simulink model "OrientationExample"  (R2024b)
settings: Solver=VariableStepAuto  StartTime=0.0  StopTime=inf  RelTol=1e-3
PostLoadFcn:
  | addpath(genpath(pwd))
settings Model: Creator=JesseJabezArendse  LastModifiedBy=JesseJabezArendse

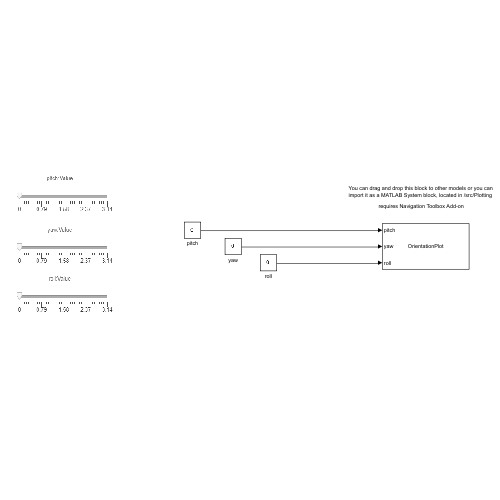
[thumbnail: Simulink's stored preview of the top-level diagram]
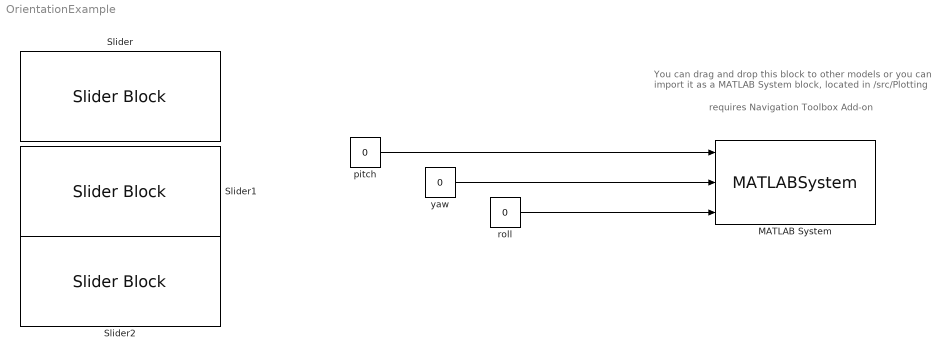
== system OrientationExample ==
  note: requires Navigation Toolbox Add-on
  note: You can drag and drop this block to other models or you can import it as a MATLAB System block, located in /src/Plotting
  MATLAB System : MATLABSystem  System=OrientationPlot
      mask Type: OrientationPlot
      mask Display:
      | disp('OrientationPlot');
      | port_label('input',1,'pitch');
      | port_label('input',2,'yaw');
      | port_label('input',3,'roll');
  Slider : SliderBlock  ScaleMax=3.14
  Slider1 : SliderBlock  ScaleMax=3.14
  Slider2 : SliderBlock  ScaleMax=3.14
  pitch : Constant  Value=0
  roll : Constant  Value=0
  yaw : Constant  Value=0
  wires:
  pitch/1 -> MATLAB System/1
  roll/1 -> MATLAB System/3
  yaw/1 -> MATLAB System/2
